simulink model "heli_q8"  (R2015b)
settings: Solver=ode1  StartTime=0.0  StopTime=inf  FixedStep=0.002  RelTol=1e-3
PostLoadFcn:
  | qc_set_target_type(getConfigSet(bdroot, 'QUARC Default Target Configuration'));
values from neighbouring files (symbols this model uses):
  calibrate_time = 2    [init_heli_day2_task3.m]
  elevation_test = 0    [init_heli_day2_task2.m]    (also in init_heli_day2_task3.m)
  F = [ K(1,1) K(1,3); K(2,1) K(2,3)]    [init_heli_day2_task2.m]    (also in init_heli_day2_task3.m)
  Joystick_gain_x = 1    [init_heli_day2_task2.m]    (also in init_heli_day2_task3.m = 0.75)
  Joystick_gain_y = 1    [init_heli_day2_task2.m]    (also in init_heli_day2_task3.m = 0.75)
  K = place(A, B, p)    [init_heli_day2_task2.m]    (also in init_heli_day2_task3.m = lqr(A, B, Q, R))
  pitch_test = 1    [init_heli_day2_task2.m]    (also in init_heli_day2_task3.m)
undefined symbols (not defined in the file or in its folder): HIL, qc_get_step_size
libraries: quarc_library x4
settings Model: SimulationMode=external  ExtModeTrigDuration=5000  Creator=Rchan  LastModifiedBy=ksteins
settings SolverCC: PositivePriorityOrder=on
settings DataIOCC: SaveFormat=Array  SignalLoggingSaveFormat=ModelDataLogs
settings OptimizationCC: ExpressionDepthLimit=2147483647  InitFltsAndDblsToZero=on
settings DebuggingCC: SaveWithParameterizedLinksMsg=none  UnderspecifiedInitializationDetection=Classic  MergeDetectMultiDrivingBlocksExec=none  SolverPrmCheckMsg=warning  MultiTaskDSMMsg=warning  MultiTaskCondExecSysMsg=none  FcnCallInpInsideContextMsg=UseLocalSettings  StateNameClashWarn=warning
settings HardwareCC: ProdBitPerPointer=32  ProdLargestAtomicFloat=None  ProdIntDivRoundTo=Undefined  ProdEndianess=Unspecified  ProdWordSize=32  ProdHWDeviceType=32-bit Generic
settings RTWCC: SystemTargetFile=quarc_win64.tlc  TemplateMakefile=quarc_default_tmf  Description=QUARC Win64 Target
settings GRTTargetCC: ParMdlRefBuildCompliant=off  CompOptLevelCompliant=off  GeneratePreprocessorConditionals=Disable all  CombineOutputUpdateFcns=off  MatFileLogging=off  GRTInterface=on  UseToolchainInfoCompliant=off  ExtMode=on  ExtModeMexFile=quarc_comm
settings ConfigComp: CovModelRefEnable=Off  CovSFcnEnable=off

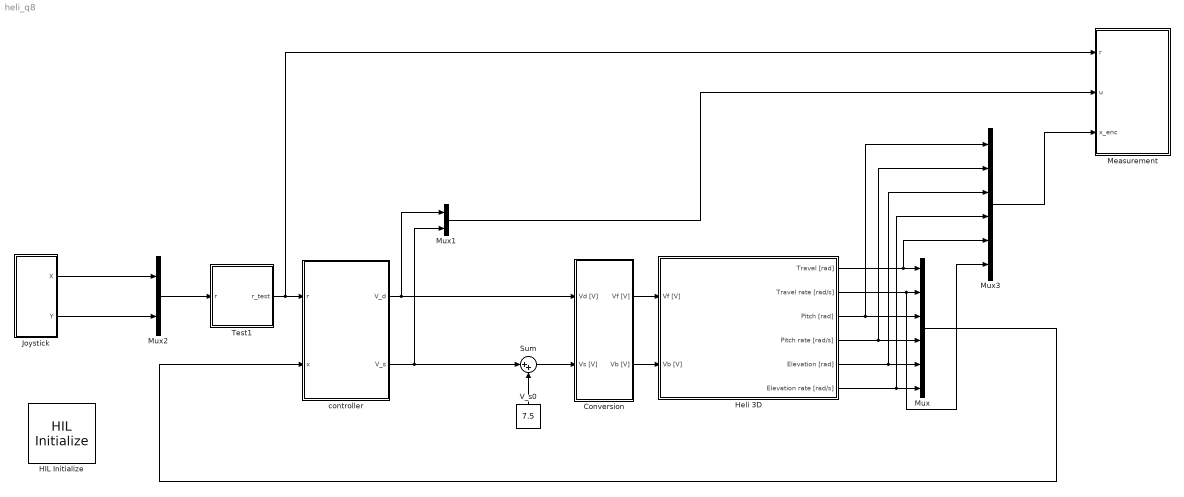
== system heli_q8 ==
  Conversion : Subsystem
  HIL Initialize : quarc_library/Data Acquisition/Generic/Configuration/HIL Initialize  Priority=-99  object_name=HIL-1  board_type=q8_usb  board_number=0  board_options=update_rate=normal;decimation=1  exclusive=off  active=off  hardware_clocks=[0:2]  clock_modes=[]  initial_clock_frequencies=[]  set_clock_params_at_start=off  set_clock_params_at_switch_in=off  set_clock_frequencies_at_start=off  set_clock_frequencies_at_switch_in=off  analog_input_channels=[0:7]  analog_input_maximums=10  analog_input_minimums=-10  set_analog_input_params_at_start=on  set_analog_input_params_at_switch_in=off  analog_output_channels=[0:7]  analog_output_maximums=10  analog_output_minimums=-10  initial_analog_outputs=[0]  final_analog_outputs=[0]  watchdog_analog_outputs=0  set_analog_output_params_at_start=on  set_analog_output_params_at_switch_in=off  set_analog_outputs_at_start=on  set_analog_outputs_at_switch_in=off  set_analog_outputs_at_terminate=on  set_analog_outputs_at_switch_out=off  set_analog_outputs_on_watchdog=off  digital_input_channels=[]  digital_output_channels=[]  digital_output_configuration=[]  initial_digital_outputs=[1]  final_digital_outputs=[1]  watchdog_digital_outputs=[1]  set_digital_output_params_at_start=off  set_digital_output_params_at_switch_in=off  set_digital_outputs_at_start=on  set_digital_outputs_at_switch_in=off  set_digital_outputs_at_terminate=on  set_digital_outputs_at_switch_out=off  set_digital_outputs_on_watchdog=off  encoder_channels=[0:7]  quadrature=[4]  encoder_filter_frequency=[]  initial_encoder_counts=[0]  set_encoder_params_at_start=on  set_encoder_params_at_switch_in=off  set_encoder_counts_at_start=on  set_encoder_counts_at_switch_in=off  pwm_channels=[0:7]  pwm_modes=0  pwm_frequency=99.532799999999995e6/4095  pwm_configuration=[0]  pwm_alignment=[0]  pwm_polarity=[1]  pwm_leading_deadband=[0]  pwm_trailing_deadband=[0]  initial_pwm_outputs=[0]  final_pwm_outputs=[0]  watchdog_pwm_outputs=[0]  set_pwm_params_at_start=on  set_pwm_params_at_switch_in=off  set_pwm_outputs_at_start=on  set_pwm_outputs_at_switch_in=off  set_pwm_outputs_at_terminate=on  set_pwm_outputs_at_switch_out=off  set_pwm_outputs_on_watchdog=off  other_output_channels=[]  initial_other_outputs=[]  final_other_outputs=[]  watchdog_other_outputs=[]  set_other_outputs_at_start=off  set_other_outputs_at_switch_in=off  set_other_outputs_at_terminate=off  set_other_outputs_at_switch_out=off  set_other_outputs_on_watchdog=off
  Heli 3D : Subsystem
  Joystick : Subsystem
  Measurement : Subsystem
  Mux : Mux  Inputs=6
  Mux1 : Mux  Inputs=2
  Mux2 : Mux  Inputs=2
  Mux3 : Mux  Inputs=6
  Sum : Sum  Inputs=|++
  Test1 : Subsystem
  V_s0 : Constant  Value=7.5
  controller : Subsystem
  wires:
  Conversion/2(Vb [V]) -> Heli 3D/2(Vb [V])
  Conversion/1(Vf [V]) -> Heli 3D/1(Vf [V])
  Heli 3D/1(Travel [rad]) -> Mux3/5, Mux/1
  Heli 3D/2(Travel rate [rad/s]) -> Mux3/6, Mux/2
  Heli 3D/3(Pitch [rad]) -> Mux3/1, Mux/3
  Heli 3D/4(Pitch rate [rad/s]) -> Mux3/2, Mux/4
  Heli 3D/6(Elevation rate [rad/s]) -> Mux3/4, Mux/6
  Heli 3D/5(Elevation [rad]) -> Mux3/3, Mux/5
  controller/2("V_s ") -> Sum/1, Mux1/2
  V_s0/1 -> Sum/2
  Sum/1 -> Conversion/2(Vs [V])
  Mux/1 -> controller/2(x)
  Joystick/1(X) -> Mux2/1
  Joystick/2(Y) -> Mux2/2
  controller/1(V_d) -> Mux1/1, Conversion/1(Vd [V])
  Mux1/1 -> Measurement/2(u)
  Mux3/1 -> Measurement/3(x_enc)
  Test1/1(r_test) -> Measurement/1(r), controller/1(r)
  Mux2/1 -> Test1/1(r)

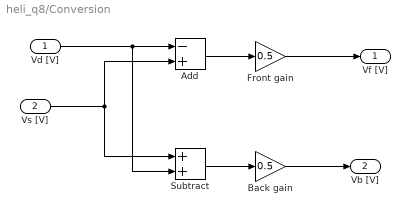
== system heli_q8/Conversion ==
  Vd [V] : Inport
  Vs [V] : Inport  Port=2
  Add : Sum  Inputs=-+
  Back gain : Gain  Gain=0.5
  Front gain : Gain  Gain=0.5
  Subtract : Sum
  Vf [V] : Outport
  Vb [V] : Outport  Port=2
  wires:
  Vd [V]/1 -> Subtract/2, Add/1
  Vs [V]/1 -> Subtract/1, Add/2
  Subtract/1 -> Back gain/1
  Back gain/1 -> Vb [V]/1
  Add/1 -> Front gain/1
  Front gain/1 -> Vf [V]/1

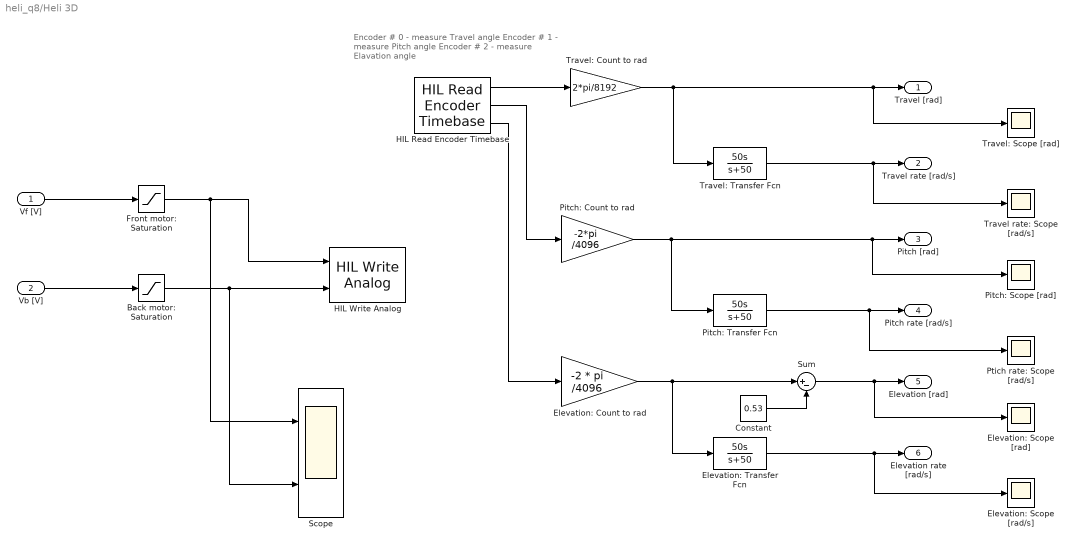
== system heli_q8/Heli 3D ==
  note: Encoder # 0 - measure Travel angle
      | Encoder # 1 - measure Pitch angle
      | Encoder # 2 - measure Elavation angle
  Vf [V] : Inport
  Vb [V] : Inport  Port=2
  Back motor: Saturation : Saturate  UpperLimit=5  LowerLimit=-5
  Constant : Constant  Value=0.53
  Elevation: Count to rad : Gain  Gain=-2 * pi /4096
  Elevation: Scope [rad/s] : Scope
  Elevation: Scope [rad] : Scope
  Elevation: Transfer Fcn : TransferFcn  Numerator=[50 0]  Denominator=[1 50]
  Front motor: Saturation : Saturate  UpperLimit=5  LowerLimit=-5
  HIL Read Encoder Timebase : quarc_library/Data Acquisition/Generic/Timebases/HIL Read Encoder Timebase  object_name=HIL-1  clock=0  channels=[0:2]  samples_in_buffer=max(ceil(1/qc_get_step_size), 1)  active=on  vector_output=off  data_type_mode=Inherit via back propagation  data_type=double
  HIL Write Analog : quarc_library/Data Acquisition/Generic/Immediate I//O/HIL Write Analog  object_name=HIL-1  channels=[0:1]  sample_time=-1  active=off  vector_input=off
  Pitch: Count to rad : Gain  Gain=-2*pi /4096
  Pitch: Scope [rad] : Scope
  Pitch: Transfer Fcn : TransferFcn  Numerator=[50 0]  Denominator=[1 50]
  Ptich rate: Scope [rad/s] : Scope
  Scope : Scope  NumInputPorts=2
  Sum : Sum  Inputs=|+-
  Travel rate: Scope [rad/s] : Scope
  Travel: Count to rad : Gain  Gain=2*pi/8192
  Travel: Scope [rad] : Scope
  Travel: Transfer Fcn : TransferFcn  Numerator=[50 0]  Denominator=[1 50]
  Travel [rad] : Outport
  Travel rate [rad/s] : Outport  Port=2
  Pitch [rad] : Outport  Port=3
  Pitch rate [rad/s] : Outport  Port=4
  Elevation [rad] : Outport  Port=5
  Elevation rate [rad/s] : Outport  Port=6
  wires:
  HIL Read Encoder Timebase/1 -> Travel: Count to rad/1
  HIL Read Encoder Timebase/2 -> Pitch: Count to rad/1
  HIL Read Encoder Timebase/3 -> Elevation: Count to rad/1
  Travel: Count to rad/1 -> Travel: Scope [rad]/1, Travel [rad]/1, Travel: Transfer Fcn/1
  Travel: Transfer Fcn/1 -> Travel rate: Scope [rad/s]/1, Travel rate [rad/s]/1
  Pitch: Count to rad/1 -> Pitch: Transfer Fcn/1, Pitch: Scope [rad]/1, Pitch [rad]/1
  Pitch: Transfer Fcn/1 -> Ptich rate: Scope [rad/s]/1, Pitch rate [rad/s]/1
  Elevation: Count to rad/1 -> Elevation: Transfer Fcn/1, Sum/1
  Elevation: Transfer Fcn/1 -> Elevation: Scope [rad/s]/1, Elevation rate [rad/s]/1
  Vf [V]/1 -> Front motor: Saturation/1
  Vb [V]/1 -> Back motor: Saturation/1
  Front motor: Saturation/1 -> Scope/1, HIL Write Analog/1
  Back motor: Saturation/1 -> Scope/2, HIL Write Analog/2
  Sum/1 -> Elevation: Scope [rad]/1, Elevation [rad]/1
  Constant/1 -> Sum/2

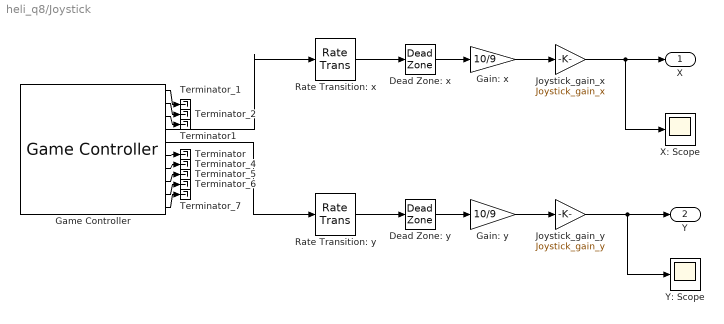
== system heli_q8/Joystick ==
  Dead Zone: x : DeadZone  LowerValue=-0.1  UpperValue=0.1  SaturateOnIntegerOverflow=on
  Dead Zone: y : DeadZone  LowerValue=-0.1  UpperValue=0.1  SaturateOnIntegerOverflow=on
  Gain: x : Gain  Gain=10/9
  Gain: y : Gain  Gain=10/9
  Game Controller : quarc_library/Devices/Peripherals/Target/Game Controller  controller=1  buffer_size=12  deadzone=[]  saturation=[]  sample_time=max(qc_get_step_size, 0.01)  auto_center=off  enabled=on
  Joystick_gain_x : Gain  Gain=Joystick_gain_x
  Joystick_gain_y : Gain  Gain=Joystick_gain_y
  Rate Transition: x : RateTransition
  Rate Transition: y : RateTransition
  Terminator : Terminator
  Terminator1 : Terminator
  Terminator_{1..2,4..7} (6 alike) : Terminator
  X: Scope : Scope
  Y: Scope : Scope
  X : Outport
  Y : Outport  Port=2
  wires:
  Rate Transition: y/1 -> Dead Zone: y/1
  Rate Transition: x/1 -> Dead Zone: x/1
  Game Controller/5 -> Rate Transition: y/1
  Game Controller/4 -> Rate Transition: x/1
  Game Controller/1 -> Terminator_1/1
  Game Controller/2 -> Terminator_2/1
  Game Controller/7 -> Terminator_4/1
  Game Controller/8 -> Terminator_5/1
  Game Controller/9 -> Terminator_6/1
  Game Controller/10 -> Terminator_7/1
  Game Controller/3 -> Terminator1/1
  Game Controller/6 -> Terminator/1
  Dead Zone: x/1 -> Gain: x/1
  Dead Zone: y/1 -> Gain: y/1
  Gain: x/1 -> Joystick_gain_x/1
  Gain: y/1 -> Joystick_gain_y/1
  Joystick_gain_x/1 -> X/1, X: Scope/1
  Joystick_gain_y/1 -> Y: Scope/1, Y/1

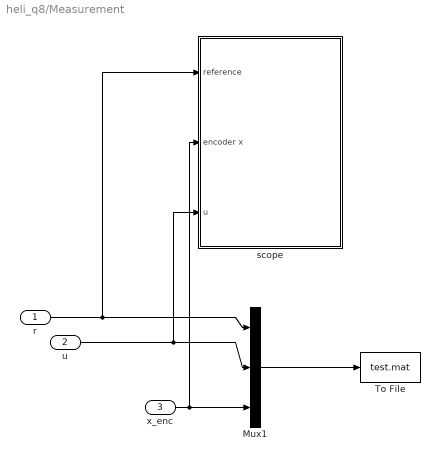
== system heli_q8/Measurement ==
  r : Inport
  u : Inport  Port=2
  x_enc : Inport  Port=3
  Mux1 : Mux  Inputs=3
  To File : ToFile  Filename=test.mat  MatrixName=data
  scope : Subsystem
  wires:
  u/1 -> scope/3(u), Mux1/2
  Mux1/1 -> To File/1
  r/1 -> scope/1(reference), Mux1/1
  x_enc/1 -> Mux1/3, scope/2(encoder x)

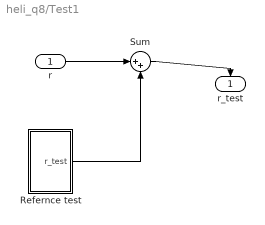
== system heli_q8/Test1 ==
  r : Inport
  Refernce test : Subsystem
  Sum : Sum  Inputs=|++
  r_test : Outport
  wires:
  Refernce test/1("r_test ") -> Sum/2
  r/1 -> Sum/1
  Sum/1 -> r_test/1

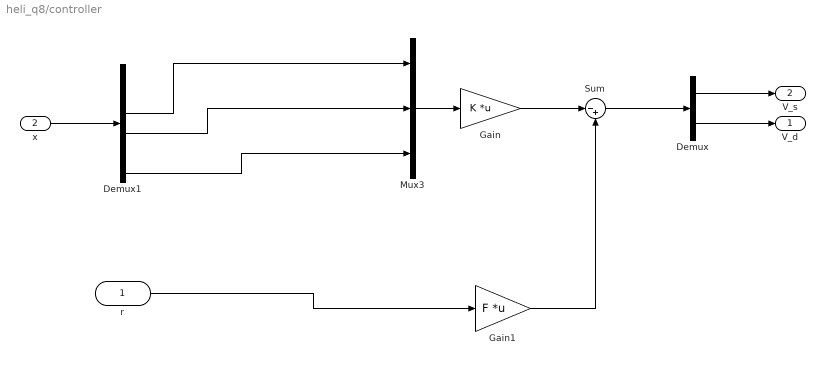
== system heli_q8/controller ==
  r : Inport
  x : Inport  Port=2
  Demux : Demux  Outputs=2
  Demux1 : Demux  Outputs=6
  Gain : Gain  Gain=K  Multiplication=Matrix(K*u)
  Gain1 : Gain  Gain=F  Multiplication=Matrix(K*u)
  Mux3 : Mux  Inputs=3
  Sum : Sum  Inputs=|-+
  V_d : Outport  InitialOutput=0
  "V_s " : Outport  Port=2  InitialOutput=0
  wires:
  x/1 -> Demux1/1
  Gain1/1 -> Sum/2
  Gain/1 -> Sum/1
  Sum/1 -> Demux/1
  Demux/2 -> V_d/1
  Demux/1 -> "V_s "/1
  Demux1/6 -> Mux3/3
  Demux1/3 -> Mux3/1
  Demux1/4 -> Mux3/2
  Mux3/1 -> Gain/1
  r/1 -> Gain1/1

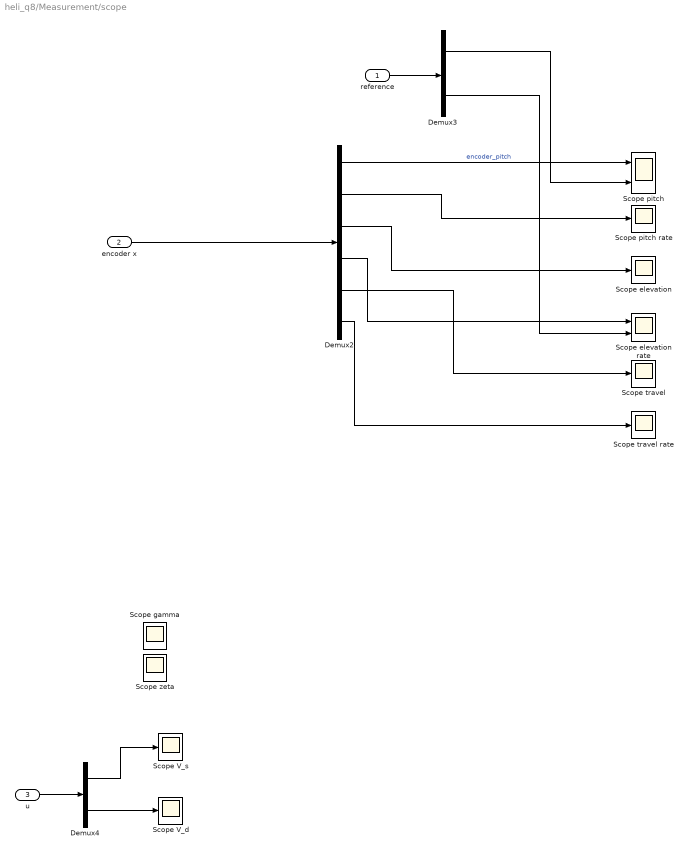
== system heli_q8/Measurement/scope ==
  reference : Inport
  encoder x : Inport  Port=2
  u : Inport  Port=3
  Demux2 : Demux  Outputs=6
  Demux3 : Demux  Outputs=2
  Demux4 : Demux  Outputs=2
  Scope V_d : Scope
  Scope V_s : Scope
  Scope elevation : Scope
  Scope elevation rate : Scope  NumInputPorts=2
  Scope gamma : Scope
  Scope pitch : Scope  NumInputPorts=2
  Scope pitch rate : Scope
  Scope travel : Scope
  Scope travel rate : Scope
  Scope zeta : Scope
  wires:
  encoder x/1 -> Demux2/1
  Demux2/4 -> Scope elevation rate/1
  Demux2/3 -> Scope elevation/1
  Demux2/2 -> Scope pitch rate/1
  Demux2/1 -> Scope pitch/1  "encoder_pitch"
  reference/1 -> Demux3/1
  Demux3/1 -> Scope pitch/2
  Demux3/2 -> Scope elevation rate/2
  Demux2/6 -> Scope travel rate/1
  u/1 -> Demux4/1
  Demux4/1 -> Scope V_s/1
  Demux4/2 -> Scope V_d/1
  Demux2/5 -> Scope travel/1

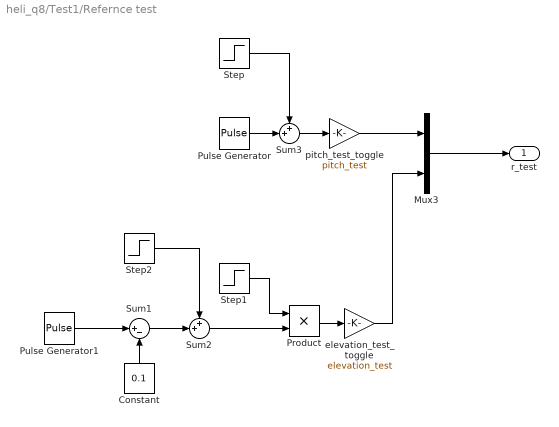
== system heli_q8/Test1/Refernce test ==
  Constant : Constant  Value=0.1
  Mux3 : Mux  Inputs=2
  Product : Product
  Pulse Generator : DiscretePulseGenerator  PulseType=Time based  Amplitude=0.5  Period=10  PulseWidth=50  PhaseDelay=5
  Pulse Generator1 : DiscretePulseGenerator  PulseType=Time based  Amplitude=0.2  Period=5  PulseWidth=50  PhaseDelay=5
  Step : Step  Time=5  After=-0.25  SampleTime=0
  Step1 : Step  Time=5  SampleTime=0
  Step2 : Step  Time=5*calibrate_time  Before=0.1  After=0  SampleTime=0
  Sum1 : Sum  Inputs=|+-
  Sum2 : Sum  Inputs=++|
  Sum3 : Sum  Inputs=++|
  elevation_test_toggle : Gain  Gain=elevation_test
  pitch_test_toggle : Gain  Gain=pitch_test
  "r_test " : Outport
  wires:
  Step/1 -> Sum3/1
  Pulse Generator/1 -> Sum3/2
  Sum3/1 -> pitch_test_toggle/1
  pitch_test_toggle/1 -> Mux3/1
  Mux3/1 -> "r_test "/1
  Product/1 -> elevation_test_toggle/1
  elevation_test_toggle/1 -> Mux3/2
  Step1/1 -> Product/1
  Pulse Generator1/1 -> Sum1/1
  Constant/1 -> Sum1/2
  Step2/1 -> Sum2/1
  Sum1/1 -> Sum2/2
  Sum2/1 -> Product/2
